simulink model "Modelo_Longitudinal_sem_Estimacao"  (R2024a)
settings: Solver=FixedStepAuto  StartTime=0.0  StopTime=10  FixedStep=10^-3  RelTol=1e-3
values from neighbouring files (symbols this model uses):
  theta = V(4)    [Eq_Mov.m]    (also in varglobal_semKF.m = 0.785398163397)
undefined symbols (not defined in the file or in its folder): sigbuilder_block
libraries: simulink_extras x1
settings Model: Creator=aluno  LastModifiedBy=wenis
settings SolverCC: AlgebraicLoopSolver=TrustRegion
settings DebuggingCC: UnconnectedInputMsg=warning  UnconnectedOutputMsg=warning  UnconnectedLineMsg=warning
settings ModelReferenceCC: EnableRefExpFcnMdlSchedulingChecks=on
settings RTWCC: GPUComputeCapability=3.5  DLArmComputeVersion=19.05

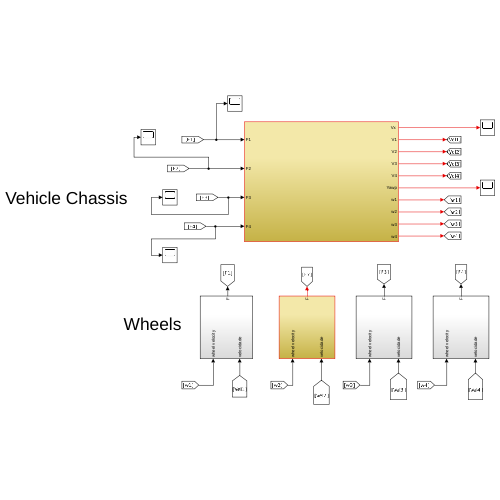
[thumbnail: Simulink's stored preview of the top-level diagram]
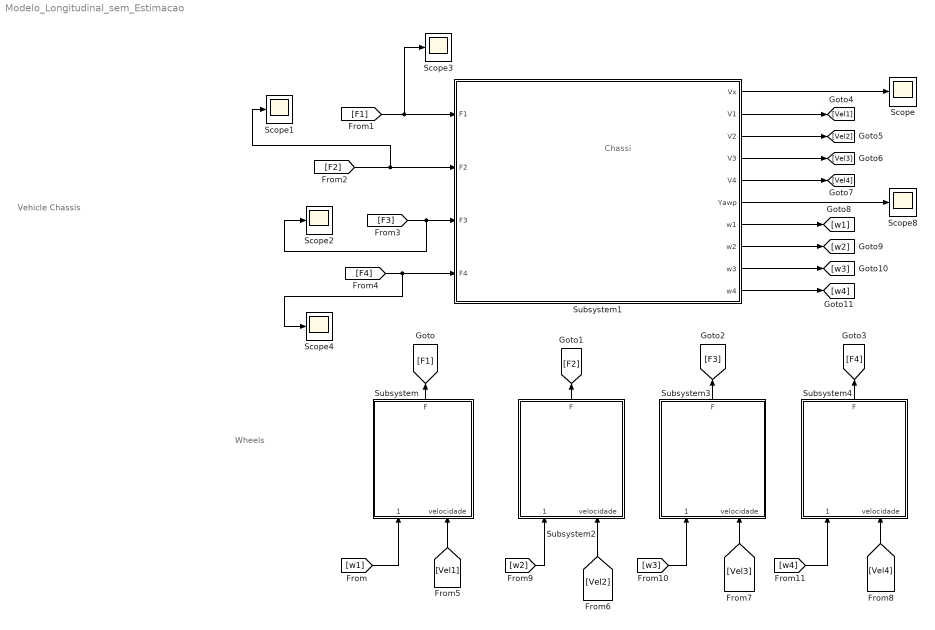
== system Modelo_Longitudinal_sem_Estimacao ==
  note: Vehicle Chassis
  note: Wheels
  note: Chassi
  Scope{,1..4,8} (6 alike) : Scope
  Subsystem : Subsystem
  Subsystem1 : Subsystem
  Subsystem2 : Subsystem
  Subsystem3 : Subsystem
  Subsystem4 : Subsystem
  wires:
  [F3] -> Subsystem1/3(F3), Scope2/1
  Subsystem4/1(F) -> [F4]
  [Vel2] -> Subsystem2/2(velocidade)
  [w1] -> Subsystem/1(wheel velocity)
  Subsystem3/1(F) -> [F3]
  [F4] -> Subsystem1/4(F4), Scope4/1
  [Vel1] -> Subsystem/2(velocidade)
  [F2] -> Subsystem1/2(F2), Scope1/1
  Subsystem/1(F) -> [F1]
  Subsystem2/1(F) -> [F2]
  [F1] -> Subsystem1/1(F1), Scope3/1
  [Vel3] -> Subsystem3/2(velocidade)
  Subsystem1/6(Yawp) -> Scope8/1
  [Vel4] -> Subsystem4/2(velocidade)
  [w2] -> Subsystem2/1(wheel velocity)
  [w3] -> Subsystem3/1(wheel velocity)
  [w4] -> Subsystem4/1(wheel velocity)
  Subsystem1/1("Vx ") -> Scope/1
  Subsystem1/2(V1) -> [Vel1]
  Subsystem1/3(V2) -> [Vel2]
  Subsystem1/4(V3) -> [Vel3]
  Subsystem1/5(V4) -> [Vel4]
  Subsystem1/7(w1) -> [w1]
  Subsystem1/8(w2) -> [w2]
  Subsystem1/9(w3) -> [w3]
  Subsystem1/10(w4) -> [w4]

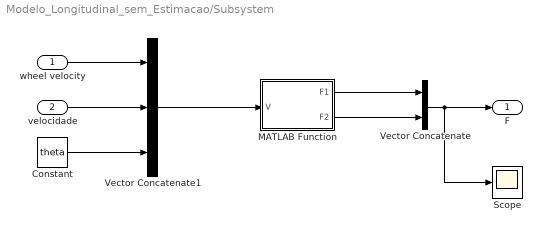
== system Modelo_Longitudinal_sem_Estimacao/Subsystem ==
  wheel velocity : Inport
  velocidade : Inport  Port=2
  Constant : Constant  Value=theta
  MATLAB Function : MATLAB Function  TreatAsAtomicUnit=on
  Scope : Scope
  Vector Concatenate : Concatenate
  Vector Concatenate1 : Concatenate  NumInputs=3
  F : Outport
  wires:
  velocidade/1 -> Vector Concatenate1/2
  Vector Concatenate/1 -> Scope/1, F/1
  wheel velocity/1 -> Vector Concatenate1/1
  Constant/1 -> Vector Concatenate1/3
  Vector Concatenate1/1 -> MATLAB Function/1(V)
  MATLAB Function/1(F1) -> Vector Concatenate/1
  MATLAB Function/2(F2) -> Vector Concatenate/2

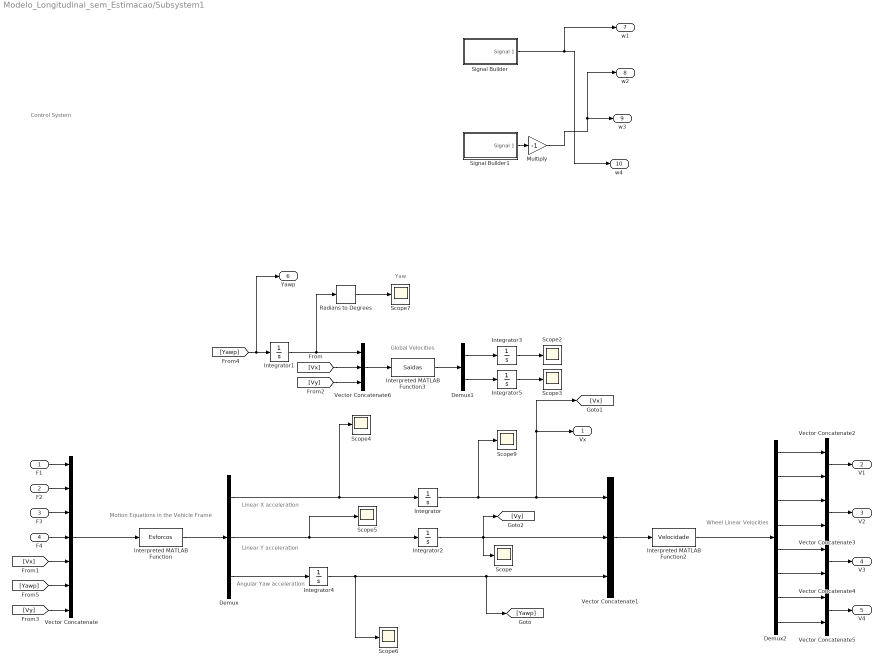
== system Modelo_Longitudinal_sem_Estimacao/Subsystem1 ==
  note: Yaw
  note: Wheel Linear Velocities
  note: Angular Yaw acceleration
  note: Linear X acceleration
  note: Motion Equations in the Vehicle Frame
  note: Global Velocities
  note: Linear Y acceleration
  note: Control System
  F1 : Inport
  F2 : Inport  Port=2
  F3 : Inport  Port=3
  F4 : Inport  Port=4
  Demux : Demux  Outputs=3
  Demux1 : Demux  Outputs=2
  Demux2 : Demux  Outputs=8
  Integrator{,1..5} (6 alike) : Integrator
  Interpreted MATLAB Function : MATLABFcn  MATLABFcn=Esforcos  OutputDimensions=3
  Interpreted MATLAB Function2 : MATLABFcn  MATLABFcn=Velocidade  OutputDimensions=8
  Interpreted MATLAB Function3 : MATLABFcn  MATLABFcn=Saidas  OutputDimensions=2
  Multiply : Gain  Gain=-1
  Radians to Degrees : simulink_extras/Transformations/Radians to Degrees
  Scope{,2..7,9} (8 alike) : Scope
  Signal Builder : Subsystem  Tag=STV Subsys  LoadFcn=sigbuilder_block('load');  StartFcn=sigbuilder_block('start');  StopFcn=sigbuilder_block('stop');  ClipboardFcn=sigbuilder_block('clipboard');  mask(Sigbuilder block){tuvar=[0:10]}
      mask help: Simulink:masks:SigbuilderBlock_MD
      mask init:
      | if ~strcmp(get_param(bdroot(gcbh),'SimulationStatus'),'stopped') tuvar = sigbuilder_block('maskInit'); end
      settings: CopyFcn=sigbuilder_block('copy');  DeleteFcn=sigbuilder_block('delete');  ModelCloseFcn=sigbuilder_block('modelClose');  PreSaveFcn=sigbuilder_block('preSave');  PauseFcn=sigbuilder_block('pause');  ContinueFcn=sigbuilder_block('continue');  NameChangeFcn=sigbuilder_block('namechange');  OpenFcn=sigbuilder_block('open',[433.5 37.5 765.75 465.75 ]);  CloseFcn=sigbuilder_block('close');
      mask Display: plot(0, 0, 100, 100,[2, 2, 32, 32, 2], [68, 8, 8, 68, 68],[32, 2], [38, 38], [32, 19, 2],[53, 60, 44], [32, 17, 17, 2],[16, 16, 31, 31]);txt = getActiveGroup(gcbh);text(2, 100, txt,'verticalAlignment', 'top');
  Signal Builder1 : Subsystem  Tag=STV Subsys  LoadFcn=sigbuilder_block('load');  StartFcn=sigbuilder_block('start');  StopFcn=sigbuilder_block('stop');  ClipboardFcn=sigbuilder_block('clipboard');  mask(Sigbuilder block){tuvar=[0:10]}
      mask help: Simulink:masks:SigbuilderBlock_MD
      mask init:
      | if ~strcmp(get_param(bdroot(gcbh),'SimulationStatus'),'stopped') tuvar = sigbuilder_block('maskInit'); end
      settings: CopyFcn=sigbuilder_block('copy');  DeleteFcn=sigbuilder_block('delete');  ModelCloseFcn=sigbuilder_block('modelClose');  PreSaveFcn=sigbuilder_block('preSave');  PauseFcn=sigbuilder_block('pause');  ContinueFcn=sigbuilder_block('continue');  NameChangeFcn=sigbuilder_block('namechange');  OpenFcn=sigbuilder_block('open',[433.5 32.25 758.25 471 ]);  CloseFcn=sigbuilder_block('close');
      mask Display: plot(0, 0, 100, 100,[2, 2, 32, 32, 2], [68, 8, 8, 68, 68],[32, 2], [38, 38], [32, 19, 2],[53, 60, 44], [32, 17, 17, 2],[16, 16, 31, 31]);txt = getActiveGroup(gcbh);text(2, 100, txt,'verticalAlignment', 'top');
  Vector Concatenate : Concatenate  NumInputs=7
  Vector Concatenate1 : Concatenate  NumInputs=3
  Vector Concatenate{2..5} (4 alike) : Concatenate
  Vector Concatenate6 : Concatenate  NumInputs=3
  "Vx " : Outport
  V1 : Outport  Port=2
  V2 : Outport  Port=3
  V3 : Outport  Port=4
  V4 : Outport  Port=5
  Yawp : Outport  Port=6
  w1 : Outport  Port=7
  w2 : Outport  Port=8
  w3 : Outport  Port=9
  w4 : Outport  Port=10
  wires:
  Interpreted MATLAB Function/1 -> Demux/1
  Vector Concatenate1/1 -> Interpreted MATLAB Function2/1
  Interpreted MATLAB Function2/1 -> Demux2/1
  Demux2/1 -> Vector Concatenate2/1
  Demux2/2 -> Vector Concatenate2/2
  Vector Concatenate2/1 -> V1/1
  Demux2/4 -> Vector Concatenate3/2
  Demux2/3 -> Vector Concatenate3/1
  Vector Concatenate3/1 -> V2/1
  Integrator1/1 -> Radians to Degrees/1, Vector Concatenate6/1
  Vector Concatenate6/1 -> Interpreted MATLAB Function3/1
  Interpreted MATLAB Function3/1 -> Demux1/1
  Demux1/1 -> Integrator3/1
  Demux1/2 -> Integrator5/1
  Integrator3/1 -> Scope2/1
  Integrator5/1 -> Scope3/1
  F1/1 -> Vector Concatenate/1
  F2/1 -> Vector Concatenate/2
  F3/1 -> Vector Concatenate/3
  F4/1 -> Vector Concatenate/4
  Demux/3 -> Integrator4/1
  Demux2/6 -> Vector Concatenate4/2
  Vector Concatenate4/1 -> V3/1
  Demux2/5 -> Vector Concatenate4/1
  Demux2/8 -> Vector Concatenate5/2
  Vector Concatenate5/1 -> V4/1
  Demux2/7 -> Vector Concatenate5/1
  [Vx] -> Vector Concatenate6/2
  [Vx] -> Vector Concatenate/5
  [Vy] -> Vector Concatenate6/3
  [Vy] -> Vector Concatenate/7
  [Yawp] -> Yawp/1, Integrator1/1
  [Yawp] -> Vector Concatenate/6
  Demux/1 -> Integrator/1, Scope4/1
  Demux/2 -> Integrator2/1, Scope5/1
  Radians to Degrees/1 -> Scope7/1
  Integrator/1 -> Scope9/1, [Vx], "Vx "/1, Vector Concatenate1/1
  Integrator4/1 -> Scope6/1, [Yawp], Vector Concatenate1/3
  Integrator2/1 -> Scope/1, Vector Concatenate1/2, [Vy]
  Signal Builder/1(Signal 1) -> w4/1, w1/1
  Signal Builder1/1(Signal 1) -> Multiply/1
  Vector Concatenate/1 -> Interpreted MATLAB Function/1
  Multiply/1 -> w3/1, w2/1

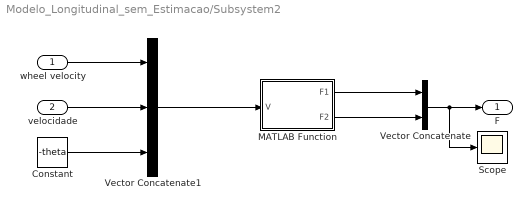
== system Modelo_Longitudinal_sem_Estimacao/Subsystem2 ==
  wheel velocity : Inport
  velocidade : Inport  Port=2
  Constant : Constant  Value=-theta
  MATLAB Function : MATLAB Function  TreatAsAtomicUnit=on
  Scope : Scope
  Vector Concatenate : Concatenate
  Vector Concatenate1 : Concatenate  NumInputs=3
  F : Outport
  wires:
  Vector Concatenate1/1 -> MATLAB Function/1(V)
  MATLAB Function/1(F1) -> Vector Concatenate/1
  MATLAB Function/2(F2) -> Vector Concatenate/2
  wheel velocity/1 -> Vector Concatenate1/1
  Constant/1 -> Vector Concatenate1/3
  velocidade/1 -> Vector Concatenate1/2
  Vector Concatenate/1 -> Scope/1, F/1

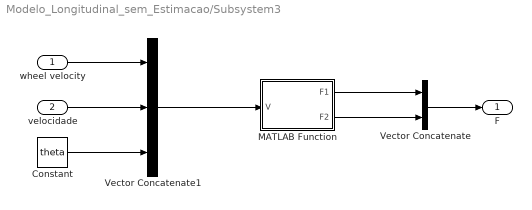
== system Modelo_Longitudinal_sem_Estimacao/Subsystem3 ==
  wheel velocity : Inport
  velocidade : Inport  Port=2
  Constant : Constant  Value=theta
  MATLAB Function : MATLAB Function  TreatAsAtomicUnit=on
  Vector Concatenate : Concatenate
  Vector Concatenate1 : Concatenate  NumInputs=3
  F : Outport
  wires:
  Vector Concatenate1/1 -> MATLAB Function/1(V)
  MATLAB Function/1(F1) -> Vector Concatenate/1
  MATLAB Function/2(F2) -> Vector Concatenate/2
  wheel velocity/1 -> Vector Concatenate1/1
  Constant/1 -> Vector Concatenate1/3
  velocidade/1 -> Vector Concatenate1/2
  Vector Concatenate/1 -> F/1

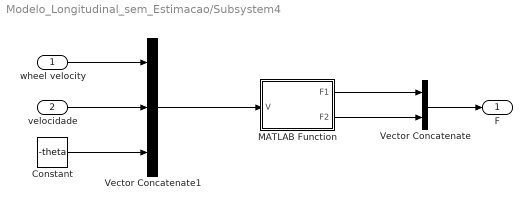
== system Modelo_Longitudinal_sem_Estimacao/Subsystem4 ==
  wheel velocity : Inport
  velocidade : Inport  Port=2
  Constant : Constant  Value=-theta
  MATLAB Function : MATLAB Function  TreatAsAtomicUnit=on
  Vector Concatenate : Concatenate
  Vector Concatenate1 : Concatenate  NumInputs=3
  F : Outport
  wires:
  Vector Concatenate1/1 -> MATLAB Function/1(V)
  MATLAB Function/1(F1) -> Vector Concatenate/1
  MATLAB Function/2(F2) -> Vector Concatenate/2
  wheel velocity/1 -> Vector Concatenate1/1
  Constant/1 -> Vector Concatenate1/3
  velocidade/1 -> Vector Concatenate1/2
  Vector Concatenate/1 -> F/1

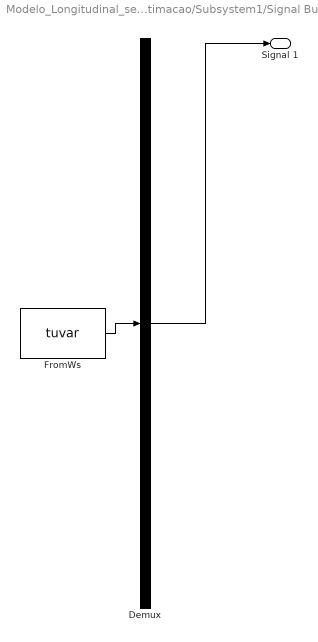
== system Modelo_Longitudinal_sem_Estimacao/Subsystem1/Signal Builder ==
  Demux : Demux  Tag=STV Demux  Outputs=1
      settings: DisplayOption=none
  FromWs : FromWorkspace  Tag=STV FromWs  VariableName=tuvar
      SigBuilderData=|
      | common.afterFinalStr = 'Extrapolate'
      | common.sampleTime = 0
      | dataSet.timeRange = [0 20]
      | dataSet.name = 'Group 1'
      | sbobj.Groups.Name = 'Group 1'
      | sbobj.Groups.Signals.Name = 'Signal 1'
      | sbobj.Groups.Signals.XData = [0 1.7 1.7 20]
      | sbobj.Groups.Signals.YData = [0 0 0.5 0.5]
      | sbobj.Groups.TimeRange = [0 20]
  Signal 1 : Outport  Tag=STV Outport
  wires:
  Demux/1 -> Signal 1/1
  FromWs/1 -> Demux/1

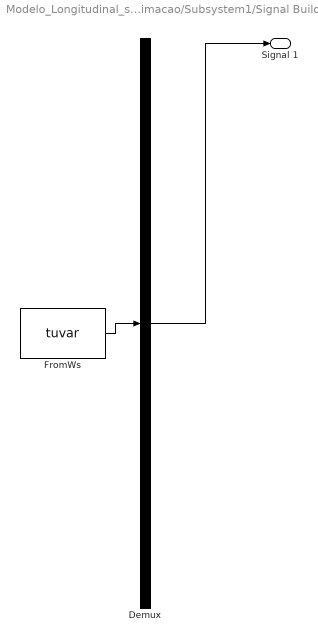
== system Modelo_Longitudinal_sem_Estimacao/Subsystem1/Signal Builder1 ==
  Demux : Demux  Tag=STV Demux  Outputs=1
      settings: DisplayOption=none
  FromWs : FromWorkspace  Tag=STV FromWs  VariableName=tuvar
      SigBuilderData=|
      | common.afterFinalStr = 'Extrapolate'
      | common.sampleTime = 0
      | dataSet.timeRange = [0 20]
      | dataSet.name = 'Group 1'
      | sbobj.Groups.Name = 'Group 1'
      | sbobj.Groups.Signals.Name = 'Signal 1'
      | sbobj.Groups.Signals.XData = [0 1.7 1.7 20]
      | sbobj.Groups.Signals.YData = [0 0 0.5 0.5]
      | sbobj.Groups.TimeRange = [0 20]
  Signal 1 : Outport  Tag=STV Outport
  wires:
  Demux/1 -> Signal 1/1
  FromWs/1 -> Demux/1

== matlab function Modelo_Longitudinal_sem_Estimacao/Subsystem/MATLAB Function ==
  data: F1 output; V input; F2 output
function [F1,F2]   =func(V)


g=9.81;
uc_x=1.0;
uc_y=0.03;
theta=pi/4;
vlimite = 0.5;
l=0.70;
w=0.50;
m=100;
Iz = (1/12)*m*(l^2+w^2);
r=0.12;

u = [uc_x;uc_y];

w = V(1);
v = [V(2);V(3)];
theta = V(4);

TF_wheel_roller = [cos(theta) -sin(theta);
                   sin(theta) cos(theta)];

Vd = -(TF_wheel_roller')*v+[w*r;0];

Fw = ((m*g/4)/(vlimite))*[Vd(1)*u(1);Vd(2)*u(2)];

F = TF_wheel_roller*Fw;
F1 = F(1);
F2 = F(2);
end

== matlab function Modelo_Longitudinal_sem_Estimacao/Subsystem3/MATLAB Function ==
  data: F1 output; V input; F2 output
function [F1,F2]   =func(V)


g=9.81;
uc_x=1.0;
uc_y=0.03;
theta=pi/4;
vlimite = 0.5;
l=0.70;
w=0.50;
m=100;
Iz = (1/12)*m*(l^2+w^2);
r=0.12;

u = [uc_x;uc_y];

w = V(1);
v = [V(2);V(3)];
theta = V(4);

TF_wheel_roller = [cos(theta) -sin(theta);
                   sin(theta) cos(theta)];

Vd = -(TF_wheel_roller')*v+[w*r;0];

Fw = ((m*g/4)/(vlimite))*[Vd(1)*u(1);Vd(2)*u(2)];

F = TF_wheel_roller*Fw;
F1 = F(1);
F2 = F(2);
end

== matlab function Modelo_Longitudinal_sem_Estimacao/Subsystem4/MATLAB Function ==
  data: F1 output; V input; F2 output
function [F1,F2]   =func(V)


g=9.81;
uc_x=1.0;
uc_y=0.03;
theta=pi/4;
vlimite = 0.5;
l=0.70;
w=0.50;
m=100;
Iz = (1/12)*m*(l^2+w^2);
r=0.12;

u = [uc_x;uc_y];

w = V(1);
v = [V(2);V(3)];
theta = V(4);

TF_wheel_roller = [cos(theta) -sin(theta);
                   sin(theta) cos(theta)];

Vd = -(TF_wheel_roller')*v+[w*r;0];

Fw = ((m*g/4)/(vlimite))*[Vd(1)*u(1);Vd(2)*u(2)];

F = TF_wheel_roller*Fw;
F1 = F(1);
F2 = F(2);
end

== matlab function Modelo_Longitudinal_sem_Estimacao/Subsystem2/MATLAB Function ==
  data: F1 output; V input; F2 output
function [F1,F2]   =func(V)


g=9.81;
uc_x=1.0;
uc_y=0.03;
theta=pi/4;
vlimite = 0.5;
l=0.70;
w=0.50;
m=100;
Iz = (1/12)*m*(l^2+w^2);
r=0.12;

u = [uc_x;uc_y];

w = V(1);
v = [V(2);V(3)];
theta = V(4);

TF_wheel_roller = [cos(theta) -sin(theta);
                   sin(theta) cos(theta)];

Vd = -(TF_wheel_roller')*v+[w*r;0];

Fw = ((m*g/4)/(vlimite))*[Vd(1)*u(1);Vd(2)*u(2)];

F = TF_wheel_roller*Fw;
F1 = F(1);
F2 = F(2);
end
